simulink model "symbol_mapping"  (R2020b)
settings: Solver=VariableStepAuto  StartTime=0.0  StopTime=10.0  RelTol=1e-3
values from neighbouring files (symbols this model uses):
  fs = 160e6    (= 160000000)    [setup.m]
libraries: hdlsllib x37
settings Model: Creator=ckb13136  LastModifiedBy=LDM

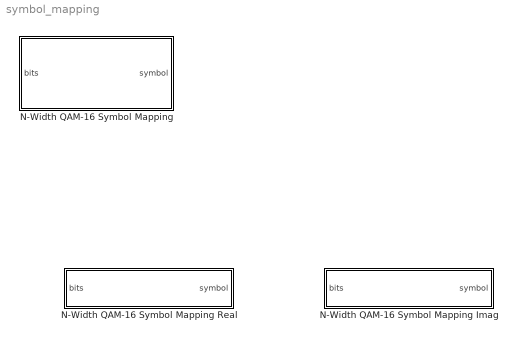
== system symbol_mapping ==
  N-Width QAM-16 Symbol Mapping : Subsystem  mask{bits=4}
      mask prompts: bits "Width:"
      mask init:
      | top_block = gcb;
      | block_names = find_system(top_block, 'LookUnderMasks','on', 'SearchDepth','1');
      | 
      | in_block = sprintf('%s/bits', top_block);
      | out_block = sprintf('%s/symbol', top_block);
      | qam_16_block = sprintf('%s/QAM-16 Symbol Mapping 0', top_block);
      | % enable_block = sprintf('%s/enable', n_qam_16);
      | 
      | keep_blocks = {top_block, in_block, out_block, qam_16_block};
      | 
      | for i = 1:length(block_names)
      |     if ~ismember(block_names{i}, keep_blocks)
      |         delete_block(block_names{i});
      |     end
      | end
      | delete_line(find_system(top_block,'LookUnderMasks', 'all','SearchDepth', '1', 'FindAll','on','type','line'));
      | 
      | % Add QAM-16 Mapping Blocks
      | pos = get_param(qam_16_block, 'position');
      | new_pos = pos;
      | set_param(qam_16_block, 'n', num2str(bits-4));
      | for bit = 4:4:bits-1
      |     new_block = sprintf('%s%d', qam_16_block(1:end-1), bit/4);
      |     add_block(qam_16_block, new_block);
      |     new_pos = pos + ([0 60 0 60] * (bit/4));
      |     set_param(new_block, 'position', new_pos);
      |     set_param(new_block, 'n', num2str(bits-4-bit));
      | end
      | 
      | % Add the Bit Concat
      | concat_block = sprintf('%s/concat', top_block);
      | add_block('hdlsllib/Logic and Bit Operations/Bit Concat', concat_block);
      | set_param(concat_block, 'numInputs', num2str(bits/2));
      | concat_position = new_pos + [175 0 175 0];
      | concat_position(2) = pos(2);
      | set_param(concat_block, 'position', concat_position);
      | 
      | % Reposition Input and Outputs
      | out_position = get_param(out_block, 'position');
      | height = out_position(4) - out_position(2);
      | width = out_position(3) - out_position(1);
      | middle_h = (concat_position(4) - concat_position(2))/2 + concat_position(2);
      | out_position = [concat_position(1) + 175, middle_h - height/2, concat_position(1) + 175 + width, middle_h + height/2];
      | set_param(out_block, 'position', out_position);
      | 
      | in_position = [concat_position(1) - 300, middle_h - height/2, concat_position(1) - 300 + width, middle_h + height/2];
      | set_param(in_block, 'position', in_position);
      | 
      | % enable_position = get_param(enable_block, 'position');
      | % set_param(enable_block, 'position', enable_position - [0 100 0 100]);
      | 
      | % Connect Ports
      | for bit = 1:4:bits
      |     add_line(top_block,'bits/1',sprintf('QAM-16 Symbol Mapping %d/1',(bit-1)/4));
      |     add_line(top_block,sprintf('QAM-16 Symbol Mapping %d/1',(bit-1)/4),sprintf('concat/%d', ceil(bit/2)));
      |     add_line(top_block,sprintf('QAM-16 Symbol Mapping %d/2',(bit-1)/4),sprintf('concat/%d', ceil(bit/2)+1));
      | end
      | add_line(top_block,'concat/1','symbol/1');
  N-Width QAM-16 Symbol Mapping Imag : Subsystem  mask{bits=64}
      mask prompts: bits "Width:"
      mask init:
      | top_block = gcb;
      | set_param(top_block, 'LinkStatus', 'none');
      | 
      | block_names = find_system(top_block, 'LookUnderMasks','on', 'SearchDepth','1');
      | 
      | in_block = sprintf('%s/bits', top_block);
      | out_block = sprintf('%s/symbol', top_block);
      | qam_16_block = sprintf('%s/QAM-16 Symbol Mapping 0', top_block);
      | % enable_block = sprintf('%s/enable', n_qam_16);
      | 
      | keep_blocks = {top_block, in_block, out_block, qam_16_block};
      | 
      | for i = 1:length(block_names)
      |     if ~ismember(block_names{i}, keep_blocks)
      |         delete_block(block_names{i});
      |     end
      | end
      | delete_line(find_system(top_block,'LookUnderMasks', 'all','SearchDepth', '1', 'FindAll','on','type','line'));
      | 
      | % Add QAM-16 Mapping Blocks
      | pos = get_param(qam_16_block, 'position');
      | new_pos = pos;
      | set_param(qam_16_block, 'n', num2str(bits-4));
      | for bit = 4:4:bits-1
      |     new_block = sprintf('%s%d', qam_16_block(1:end-1), bit/4);
      |     add_block(qam_16_block, new_block);
      |     new_pos = pos + ([0 60 0 60] * (bit/4));
      |     set_param(new_block, 'position', new_pos);
      |     set_param(new_block, 'n', num2str(bits-4-bit));
      | end
      | 
      | % Add the Bit Concat
      | concat_block = sprintf('%s/concat', top_block);
      | add_block('hdlsllib/Logic and Bit Operations/Bit Concat', concat_block);
      | set_param(concat_block, 'numInputs', num2str(bits/4));
      | concat_position = new_pos + [175 0 175 0];
      | concat_position(2) = pos(2);
      | set_param(concat_block, 'position', concat_position);
      | 
      | % Reposition Input and Outputs
      | out_position = get_param(out_block, 'position');
      | height = out_position(4) - out_position(2);
      | width = out_position(3) - out_position(1);
      | middle_h = (concat_position(4) - concat_position(2))/2 + concat_position(2);
      | out_position = [concat_position(1) + 175, middle_h - height/2, concat_position(1) + 175 + width, middle_h + height/2];
      | set_param(out_block, 'position', out_position);
      | 
      | in_position = [concat_position(1) - 300, middle_h - height/2, concat_position(1) - 300 + width, middle_h + height/2];
      | set_param(in_block, 'position', in_position);
      | 
      | % enable_position = get_param(enable_block, 'position');
      | % set_param(enable_block, 'position', enable_position - [0 100 0 100]);
      | 
      | % Connect Ports
      | for bit = 1:4:bits
      |     add_line(top_block,'bits/1',sprintf('QAM-16 Symbol Mapping %d/1',(bit-1)/4));
      |     add_line(top_block,sprintf('QAM-16 Symbol Mapping %d/1',(bit-1)/4),sprintf('concat/%d', ceil(bit/4)));
      | %     add_line(top_block,sprintf('QAM-16 Symbol Mapping %d/2',(bit-1)/4),sprintf('concat/%d', ceil(bit/2)+1));
      | end
      | add_line(top_block,'concat/1','symbol/1');
  N-Width QAM-16 Symbol Mapping Real : Subsystem  mask{bits=64}
      mask prompts: bits "Width:"
      mask init: same as symbol_mapping/N-Width QAM-16 Symbol Mapping Imag

== system symbol_mapping/N-Width QAM-16 Symbol Mapping ==
  bits : Inport
  QAM-16 Symbol Mapping 0 : Subsystem  mask{n=0}
  concat : hdlsllib/Logic and Bit Operations/Bit Concat  numInputs=2
  symbol : Outport
  wires:
  bits/1 -> QAM-16 Symbol Mapping 0/1(bits)
  QAM-16 Symbol Mapping 0/1(Q) -> concat/1
  QAM-16 Symbol Mapping 0/2(I) -> concat/2
  concat/1 -> symbol/1

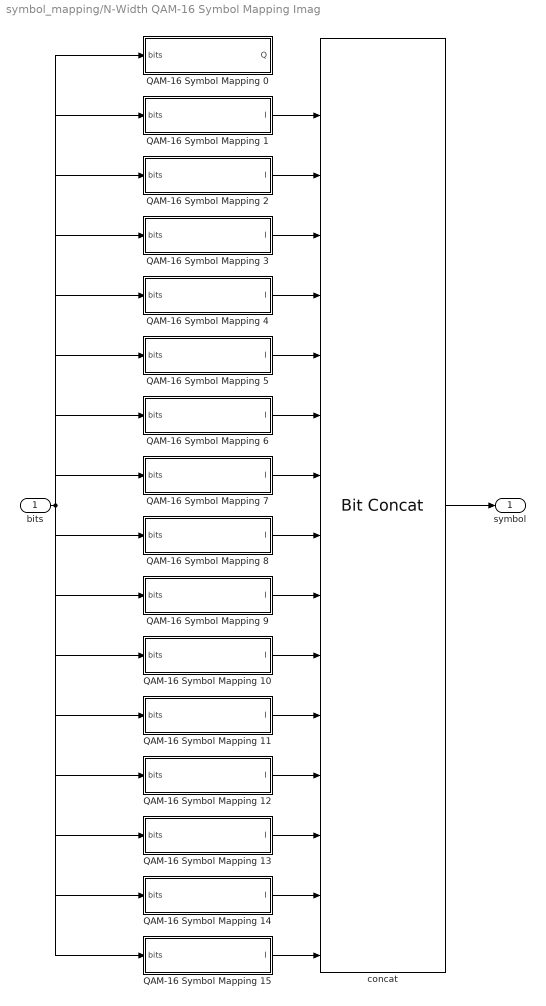
== system symbol_mapping/N-Width QAM-16 Symbol Mapping Imag ==
  bits : Inport
  QAM-16 Symbol Mapping 0 : Subsystem  mask{n=0}
  QAM-16 Symbol Mapping 1 : Subsystem  mask{n=56}
  QAM-16 Symbol Mapping 10 : Subsystem  mask{n=20}
  QAM-16 Symbol Mapping 11 : Subsystem  mask{n=16}
  QAM-16 Symbol Mapping 12 : Subsystem  mask{n=12}
  QAM-16 Symbol Mapping 13 : Subsystem  mask{n=8}
  QAM-16 Symbol Mapping 14 : Subsystem  mask{n=4}
  QAM-16 Symbol Mapping 15 : Subsystem  mask{n=0}
  QAM-16 Symbol Mapping 2 : Subsystem  mask{n=52}
  QAM-16 Symbol Mapping 3 : Subsystem  mask{n=48}
  QAM-16 Symbol Mapping 4 : Subsystem  mask{n=44}
  QAM-16 Symbol Mapping 5 : Subsystem  mask{n=40}
  QAM-16 Symbol Mapping 6 : Subsystem  mask{n=36}
  QAM-16 Symbol Mapping 7 : Subsystem  mask{n=32}
  QAM-16 Symbol Mapping 8 : Subsystem  mask{n=28}
  QAM-16 Symbol Mapping 9 : Subsystem  mask{n=24}
  concat : hdlsllib/Logic and Bit Operations/Bit Concat  numInputs=16
  symbol : Outport
  wires:
  bits/1 -> QAM-16 Symbol Mapping 0/1(bits), QAM-16 Symbol Mapping 1/1(bits), QAM-16 Symbol Mapping 2/1(bits), QAM-16 Symbol Mapping 3/1(bits), QAM-16 Symbol Mapping 4/1(bits), QAM-16 Symbol Mapping 5/1(bits), QAM-16 Symbol Mapping 6/1(bits), QAM-16 Symbol Mapping 7/1(bits), QAM-16 Symbol Mapping 8/1(bits), QAM-16 Symbol Mapping 9/1(bits), QAM-16 Symbol Mapping 10/1(bits), QAM-16 Symbol Mapping 11/1(bits), QAM-16 Symbol Mapping 12/1(bits), QAM-16 Symbol Mapping 13/1(bits), QAM-16 Symbol Mapping 14/1(bits), QAM-16 Symbol Mapping 15/1(bits)
  ? -> concat/1
  QAM-16 Symbol Mapping 1/1(I) -> concat/2
  QAM-16 Symbol Mapping 2/1(I) -> concat/3
  QAM-16 Symbol Mapping 3/1(I) -> concat/4
  QAM-16 Symbol Mapping 4/1(I) -> concat/5
  QAM-16 Symbol Mapping 5/1(I) -> concat/6
  QAM-16 Symbol Mapping 6/1(I) -> concat/7
  QAM-16 Symbol Mapping 7/1(I) -> concat/8
  QAM-16 Symbol Mapping 8/1(I) -> concat/9
  QAM-16 Symbol Mapping 9/1(I) -> concat/10
  QAM-16 Symbol Mapping 10/1(I) -> concat/11
  QAM-16 Symbol Mapping 11/1(I) -> concat/12
  QAM-16 Symbol Mapping 12/1(I) -> concat/13
  QAM-16 Symbol Mapping 13/1(I) -> concat/14
  QAM-16 Symbol Mapping 14/1(I) -> concat/15
  QAM-16 Symbol Mapping 15/1(I) -> concat/16
  concat/1 -> symbol/1

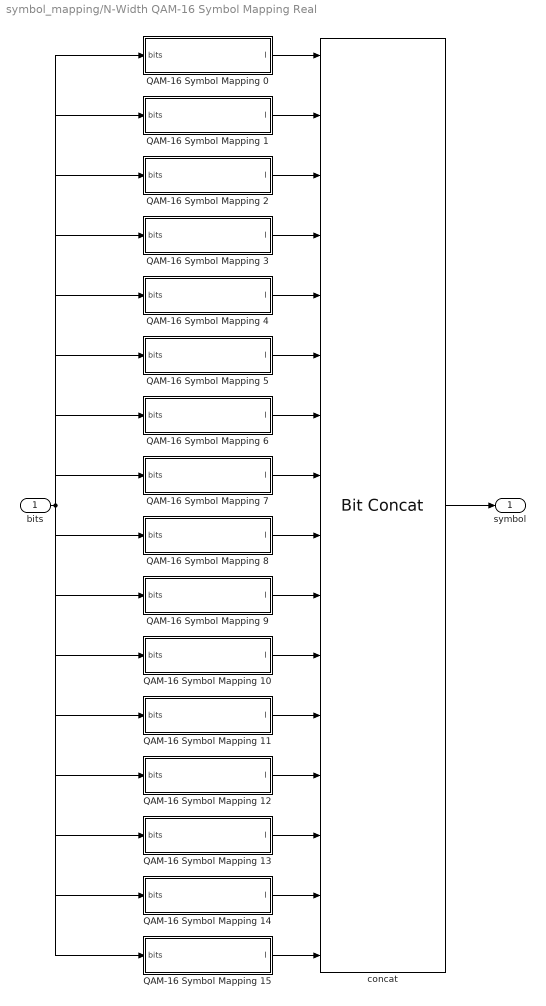
== system symbol_mapping/N-Width QAM-16 Symbol Mapping Real ==
  bits : Inport
  QAM-16 Symbol Mapping 0 : Subsystem  mask{n=60}
  QAM-16 Symbol Mapping 1 : Subsystem  mask{n=56}
  QAM-16 Symbol Mapping 10 : Subsystem  mask{n=20}
  QAM-16 Symbol Mapping 11 : Subsystem  mask{n=16}
  QAM-16 Symbol Mapping 12 : Subsystem  mask{n=12}
  QAM-16 Symbol Mapping 13 : Subsystem  mask{n=8}
  QAM-16 Symbol Mapping 14 : Subsystem  mask{n=4}
  QAM-16 Symbol Mapping 15 : Subsystem  mask{n=0}
  QAM-16 Symbol Mapping 2 : Subsystem  mask{n=52}
  QAM-16 Symbol Mapping 3 : Subsystem  mask{n=48}
  QAM-16 Symbol Mapping 4 : Subsystem  mask{n=44}
  QAM-16 Symbol Mapping 5 : Subsystem  mask{n=40}
  QAM-16 Symbol Mapping 6 : Subsystem  mask{n=36}
  QAM-16 Symbol Mapping 7 : Subsystem  mask{n=32}
  QAM-16 Symbol Mapping 8 : Subsystem  mask{n=28}
  QAM-16 Symbol Mapping 9 : Subsystem  mask{n=24}
  concat : hdlsllib/Logic and Bit Operations/Bit Concat  numInputs=16
  symbol : Outport
  wires:
  bits/1 -> QAM-16 Symbol Mapping 0/1(bits), QAM-16 Symbol Mapping 1/1(bits), QAM-16 Symbol Mapping 2/1(bits), QAM-16 Symbol Mapping 3/1(bits), QAM-16 Symbol Mapping 4/1(bits), QAM-16 Symbol Mapping 5/1(bits), QAM-16 Symbol Mapping 6/1(bits), QAM-16 Symbol Mapping 7/1(bits), QAM-16 Symbol Mapping 8/1(bits), QAM-16 Symbol Mapping 9/1(bits), QAM-16 Symbol Mapping 10/1(bits), QAM-16 Symbol Mapping 11/1(bits), QAM-16 Symbol Mapping 12/1(bits), QAM-16 Symbol Mapping 13/1(bits), QAM-16 Symbol Mapping 14/1(bits), QAM-16 Symbol Mapping 15/1(bits)
  QAM-16 Symbol Mapping 0/1(I) -> concat/1
  QAM-16 Symbol Mapping 1/1(I) -> concat/2
  QAM-16 Symbol Mapping 2/1(I) -> concat/3
  QAM-16 Symbol Mapping 3/1(I) -> concat/4
  QAM-16 Symbol Mapping 4/1(I) -> concat/5
  QAM-16 Symbol Mapping 5/1(I) -> concat/6
  QAM-16 Symbol Mapping 6/1(I) -> concat/7
  QAM-16 Symbol Mapping 7/1(I) -> concat/8
  QAM-16 Symbol Mapping 8/1(I) -> concat/9
  QAM-16 Symbol Mapping 9/1(I) -> concat/10
  QAM-16 Symbol Mapping 10/1(I) -> concat/11
  QAM-16 Symbol Mapping 11/1(I) -> concat/12
  QAM-16 Symbol Mapping 12/1(I) -> concat/13
  QAM-16 Symbol Mapping 13/1(I) -> concat/14
  QAM-16 Symbol Mapping 14/1(I) -> concat/15
  QAM-16 Symbol Mapping 15/1(I) -> concat/16
  concat/1 -> symbol/1

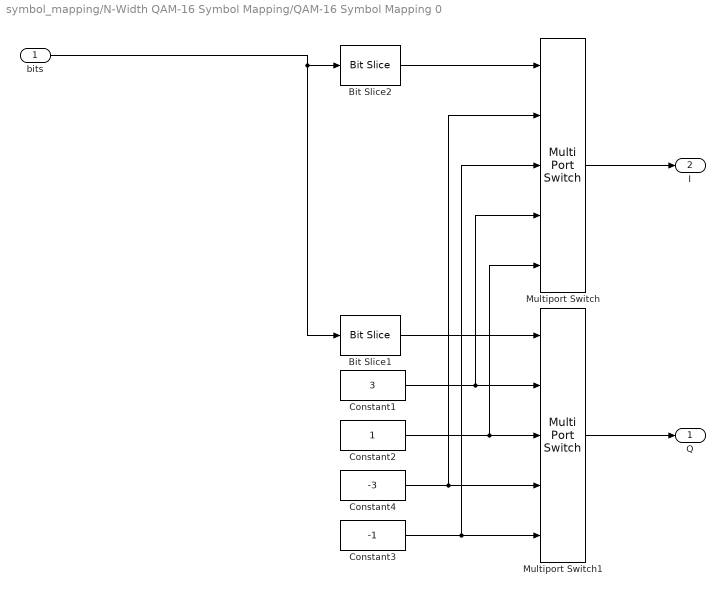
== system symbol_mapping/N-Width QAM-16 Symbol Mapping/QAM-16 Symbol Mapping 0 ==
  bits : Inport
  Bit Slice1 : hdlsllib/Logic and Bit Operations/Bit Slice  lidx=n+1  ridx=n
      settings: SourceProductBaseCode=SL
  Bit Slice2 : hdlsllib/Logic and Bit Operations/Bit Slice  lidx=n+3  ridx=n+2
      settings: SourceProductBaseCode=SL
  Constant1 : Constant  Value=3  OutDataTypeStr=fixdt(1,3,0)  SampleTime=1/(4*fs)
  Constant2 : Constant  OutDataTypeStr=fixdt(1,3,0)  SampleTime=1/(4*fs)
  Constant3 : Constant  Value=-1  OutDataTypeStr=fixdt(1,3,0)  SampleTime=1/(4*fs)
  Constant4 : Constant  Value=-3  OutDataTypeStr=fixdt(1,3,0)  SampleTime=1/(4*fs)
  Multiport Switch : MultiPortSwitch  DataPortOrder=Zero-based contiguous  Inputs=4  zeroidx=on
  Multiport Switch1 : MultiPortSwitch  DataPortOrder=Zero-based contiguous  Inputs=4  zeroidx=on
  Q : Outport
  I : Outport  Port=2
  wires:
  Bit Slice1/1 -> Multiport Switch1/1
  Multiport Switch1/1 -> Q/1
  Bit Slice2/1 -> Multiport Switch/1
  bits/1 -> Bit Slice1/1, Bit Slice2/1
  Constant3/1 -> Multiport Switch/3, Multiport Switch1/5
  Constant4/1 -> Multiport Switch/2, Multiport Switch1/4
  Constant1/1 -> Multiport Switch/4, Multiport Switch1/2
  Constant2/1 -> Multiport Switch/5, Multiport Switch1/3
  Multiport Switch/1 -> I/1

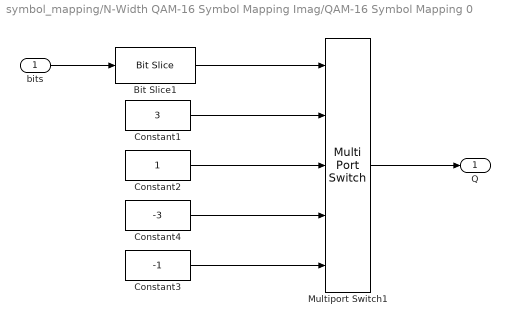
== system symbol_mapping/N-Width QAM-16 Symbol Mapping Imag/QAM-16 Symbol Mapping 0 ==
  bits : Inport
  Bit Slice1 : hdlsllib/Logic and Bit Operations/Bit Slice  lidx=n+1  ridx=n
      settings: SourceProductBaseCode=SL
  Constant1 : Constant  Value=3  OutDataTypeStr=fixdt(1,3,0)  SampleTime=1/(4*fs)
  Constant2 : Constant  OutDataTypeStr=fixdt(1,3,0)  SampleTime=1/(4*fs)
  Constant3 : Constant  Value=-1  OutDataTypeStr=fixdt(1,3,0)  SampleTime=1/(4*fs)
  Constant4 : Constant  Value=-3  OutDataTypeStr=fixdt(1,3,0)  SampleTime=1/(4*fs)
  Multiport Switch1 : MultiPortSwitch  DataPortOrder=Zero-based contiguous  Inputs=4  zeroidx=on
  Q : Outport
  wires:
  Bit Slice1/1 -> Multiport Switch1/1
  Multiport Switch1/1 -> Q/1
  bits/1 -> Bit Slice1/1
  Constant3/1 -> Multiport Switch1/5
  Constant4/1 -> Multiport Switch1/4
  Constant1/1 -> Multiport Switch1/2
  Constant2/1 -> Multiport Switch1/3

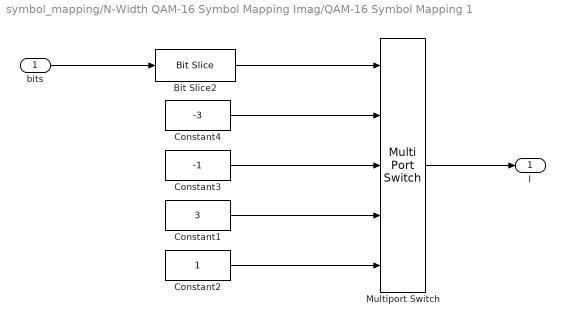
== system symbol_mapping/N-Width QAM-16 Symbol Mapping Imag/QAM-16 Symbol Mapping 1 ==
  bits : Inport
  Bit Slice2 : hdlsllib/Logic and Bit Operations/Bit Slice  lidx=n+3  ridx=n+2
      settings: SourceProductBaseCode=SL
  Constant1 : Constant  Value=3  OutDataTypeStr=fixdt(1,3,0)  SampleTime=-1
  Constant2 : Constant  OutDataTypeStr=fixdt(1,3,0)  SampleTime=-1
  Constant3 : Constant  Value=-1  OutDataTypeStr=fixdt(1,3,0)  SampleTime=-1
  Constant4 : Constant  Value=-3  OutDataTypeStr=fixdt(1,3,0)  SampleTime=-1
  Multiport Switch : MultiPortSwitch  DataPortOrder=Zero-based contiguous  Inputs=4  zeroidx=on
  I : Outport
  wires:
  Bit Slice2/1 -> Multiport Switch/1
  bits/1 -> Bit Slice2/1
  Constant3/1 -> Multiport Switch/3
  Constant4/1 -> Multiport Switch/2
  Constant1/1 -> Multiport Switch/4
  Constant2/1 -> Multiport Switch/5
  Multiport Switch/1 -> I/1

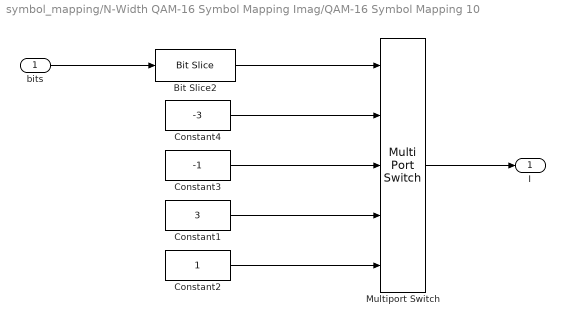
== system symbol_mapping/N-Width QAM-16 Symbol Mapping Imag/QAM-16 Symbol Mapping 10 ==
  bits : Inport
  Bit Slice2 : hdlsllib/Logic and Bit Operations/Bit Slice  lidx=n+3  ridx=n+2
      settings: SourceProductBaseCode=SL
  Constant1 : Constant  Value=3  OutDataTypeStr=fixdt(1,3,0)  SampleTime=-1
  Constant2 : Constant  OutDataTypeStr=fixdt(1,3,0)  SampleTime=-1
  Constant3 : Constant  Value=-1  OutDataTypeStr=fixdt(1,3,0)  SampleTime=-1
  Constant4 : Constant  Value=-3  OutDataTypeStr=fixdt(1,3,0)  SampleTime=-1
  Multiport Switch : MultiPortSwitch  DataPortOrder=Zero-based contiguous  Inputs=4  zeroidx=on
  I : Outport
  wires:
  Bit Slice2/1 -> Multiport Switch/1
  bits/1 -> Bit Slice2/1
  Constant3/1 -> Multiport Switch/3
  Constant4/1 -> Multiport Switch/2
  Constant1/1 -> Multiport Switch/4
  Constant2/1 -> Multiport Switch/5
  Multiport Switch/1 -> I/1

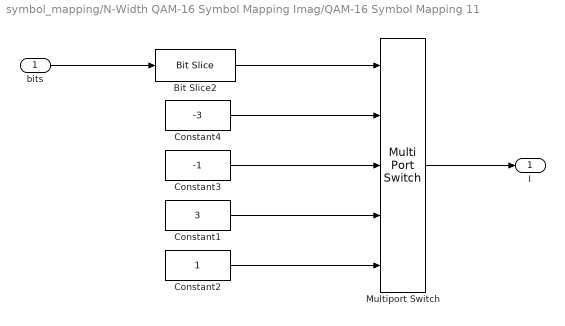
== system symbol_mapping/N-Width QAM-16 Symbol Mapping Imag/QAM-16 Symbol Mapping 11 ==
  bits : Inport
  Bit Slice2 : hdlsllib/Logic and Bit Operations/Bit Slice  lidx=n+3  ridx=n+2
      settings: SourceProductBaseCode=SL
  Constant1 : Constant  Value=3  OutDataTypeStr=fixdt(1,3,0)  SampleTime=-1
  Constant2 : Constant  OutDataTypeStr=fixdt(1,3,0)  SampleTime=-1
  Constant3 : Constant  Value=-1  OutDataTypeStr=fixdt(1,3,0)  SampleTime=-1
  Constant4 : Constant  Value=-3  OutDataTypeStr=fixdt(1,3,0)  SampleTime=-1
  Multiport Switch : MultiPortSwitch  DataPortOrder=Zero-based contiguous  Inputs=4  zeroidx=on
  I : Outport
  wires:
  Bit Slice2/1 -> Multiport Switch/1
  bits/1 -> Bit Slice2/1
  Constant3/1 -> Multiport Switch/3
  Constant4/1 -> Multiport Switch/2
  Constant1/1 -> Multiport Switch/4
  Constant2/1 -> Multiport Switch/5
  Multiport Switch/1 -> I/1

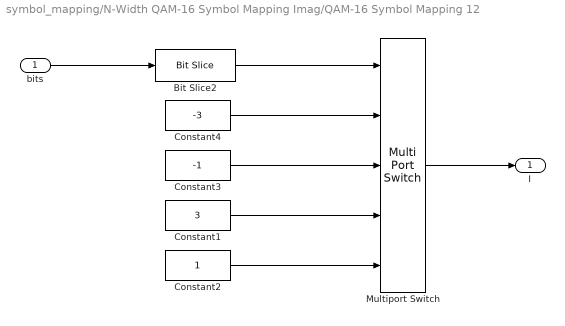
== system symbol_mapping/N-Width QAM-16 Symbol Mapping Imag/QAM-16 Symbol Mapping 12 ==
  bits : Inport
  Bit Slice2 : hdlsllib/Logic and Bit Operations/Bit Slice  lidx=n+3  ridx=n+2
      settings: SourceProductBaseCode=SL
  Constant1 : Constant  Value=3  OutDataTypeStr=fixdt(1,3,0)  SampleTime=-1
  Constant2 : Constant  OutDataTypeStr=fixdt(1,3,0)  SampleTime=-1
  Constant3 : Constant  Value=-1  OutDataTypeStr=fixdt(1,3,0)  SampleTime=-1
  Constant4 : Constant  Value=-3  OutDataTypeStr=fixdt(1,3,0)  SampleTime=-1
  Multiport Switch : MultiPortSwitch  DataPortOrder=Zero-based contiguous  Inputs=4  zeroidx=on
  I : Outport
  wires:
  Bit Slice2/1 -> Multiport Switch/1
  bits/1 -> Bit Slice2/1
  Constant3/1 -> Multiport Switch/3
  Constant4/1 -> Multiport Switch/2
  Constant1/1 -> Multiport Switch/4
  Constant2/1 -> Multiport Switch/5
  Multiport Switch/1 -> I/1

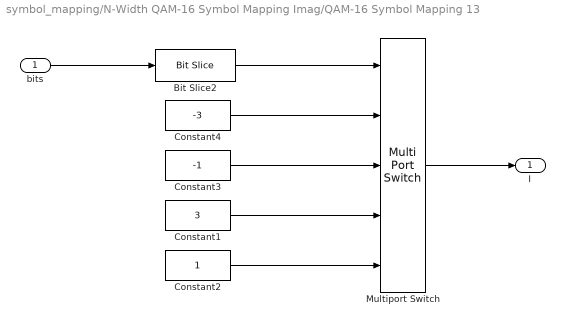
== system symbol_mapping/N-Width QAM-16 Symbol Mapping Imag/QAM-16 Symbol Mapping 13 ==
  bits : Inport
  Bit Slice2 : hdlsllib/Logic and Bit Operations/Bit Slice  lidx=n+3  ridx=n+2
      settings: SourceProductBaseCode=SL
  Constant1 : Constant  Value=3  OutDataTypeStr=fixdt(1,3,0)  SampleTime=-1
  Constant2 : Constant  OutDataTypeStr=fixdt(1,3,0)  SampleTime=-1
  Constant3 : Constant  Value=-1  OutDataTypeStr=fixdt(1,3,0)  SampleTime=-1
  Constant4 : Constant  Value=-3  OutDataTypeStr=fixdt(1,3,0)  SampleTime=-1
  Multiport Switch : MultiPortSwitch  DataPortOrder=Zero-based contiguous  Inputs=4  zeroidx=on
  I : Outport
  wires:
  Bit Slice2/1 -> Multiport Switch/1
  bits/1 -> Bit Slice2/1
  Constant3/1 -> Multiport Switch/3
  Constant4/1 -> Multiport Switch/2
  Constant1/1 -> Multiport Switch/4
  Constant2/1 -> Multiport Switch/5
  Multiport Switch/1 -> I/1

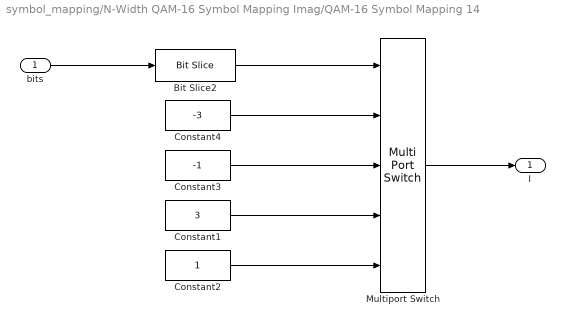
== system symbol_mapping/N-Width QAM-16 Symbol Mapping Imag/QAM-16 Symbol Mapping 14 ==
  bits : Inport
  Bit Slice2 : hdlsllib/Logic and Bit Operations/Bit Slice  lidx=n+3  ridx=n+2
      settings: SourceProductBaseCode=SL
  Constant1 : Constant  Value=3  OutDataTypeStr=fixdt(1,3,0)  SampleTime=-1
  Constant2 : Constant  OutDataTypeStr=fixdt(1,3,0)  SampleTime=-1
  Constant3 : Constant  Value=-1  OutDataTypeStr=fixdt(1,3,0)  SampleTime=-1
  Constant4 : Constant  Value=-3  OutDataTypeStr=fixdt(1,3,0)  SampleTime=-1
  Multiport Switch : MultiPortSwitch  DataPortOrder=Zero-based contiguous  Inputs=4  zeroidx=on
  I : Outport
  wires:
  Bit Slice2/1 -> Multiport Switch/1
  bits/1 -> Bit Slice2/1
  Constant3/1 -> Multiport Switch/3
  Constant4/1 -> Multiport Switch/2
  Constant1/1 -> Multiport Switch/4
  Constant2/1 -> Multiport Switch/5
  Multiport Switch/1 -> I/1

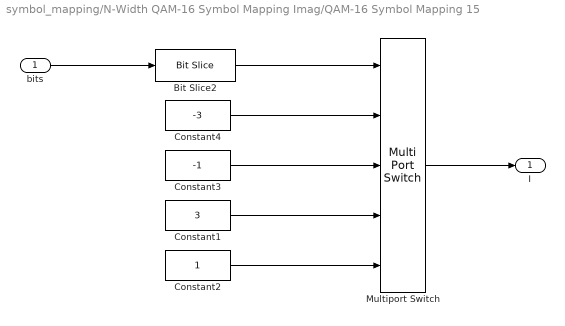
== system symbol_mapping/N-Width QAM-16 Symbol Mapping Imag/QAM-16 Symbol Mapping 15 ==
  bits : Inport
  Bit Slice2 : hdlsllib/Logic and Bit Operations/Bit Slice  lidx=n+3  ridx=n+2
      settings: SourceProductBaseCode=SL
  Constant1 : Constant  Value=3  OutDataTypeStr=fixdt(1,3,0)  SampleTime=-1
  Constant2 : Constant  OutDataTypeStr=fixdt(1,3,0)  SampleTime=-1
  Constant3 : Constant  Value=-1  OutDataTypeStr=fixdt(1,3,0)  SampleTime=-1
  Constant4 : Constant  Value=-3  OutDataTypeStr=fixdt(1,3,0)  SampleTime=-1
  Multiport Switch : MultiPortSwitch  DataPortOrder=Zero-based contiguous  Inputs=4  zeroidx=on
  I : Outport
  wires:
  Bit Slice2/1 -> Multiport Switch/1
  bits/1 -> Bit Slice2/1
  Constant3/1 -> Multiport Switch/3
  Constant4/1 -> Multiport Switch/2
  Constant1/1 -> Multiport Switch/4
  Constant2/1 -> Multiport Switch/5
  Multiport Switch/1 -> I/1

== system symbol_mapping/N-Width QAM-16 Symbol Mapping Imag/QAM-16 Symbol Mapping 2 ==
  bits : Inport
  Bit Slice2 : hdlsllib/Logic and Bit Operations/Bit Slice  lidx=n+3  ridx=n+2
      settings: SourceProductBaseCode=SL
  Constant1 : Constant  Value=3  OutDataTypeStr=fixdt(1,3,0)  SampleTime=-1
  Constant2 : Constant  OutDataTypeStr=fixdt(1,3,0)  SampleTime=-1
  Constant3 : Constant  Value=-1  OutDataTypeStr=fixdt(1,3,0)  SampleTime=-1
  Constant4 : Constant  Value=-3  OutDataTypeStr=fixdt(1,3,0)  SampleTime=-1
  Multiport Switch : MultiPortSwitch  DataPortOrder=Zero-based contiguous  Inputs=4  zeroidx=on
  I : Outport
  wires:
  Bit Slice2/1 -> Multiport Switch/1
  bits/1 -> Bit Slice2/1
  Constant3/1 -> Multiport Switch/3
  Constant4/1 -> Multiport Switch/2
  Constant1/1 -> Multiport Switch/4
  Constant2/1 -> Multiport Switch/5
  Multiport Switch/1 -> I/1

== system symbol_mapping/N-Width QAM-16 Symbol Mapping Imag/QAM-16 Symbol Mapping 3 ==
  bits : Inport
  Bit Slice2 : hdlsllib/Logic and Bit Operations/Bit Slice  lidx=n+3  ridx=n+2
      settings: SourceProductBaseCode=SL
  Constant1 : Constant  Value=3  OutDataTypeStr=fixdt(1,3,0)  SampleTime=-1
  Constant2 : Constant  OutDataTypeStr=fixdt(1,3,0)  SampleTime=-1
  Constant3 : Constant  Value=-1  OutDataTypeStr=fixdt(1,3,0)  SampleTime=-1
  Constant4 : Constant  Value=-3  OutDataTypeStr=fixdt(1,3,0)  SampleTime=-1
  Multiport Switch : MultiPortSwitch  DataPortOrder=Zero-based contiguous  Inputs=4  zeroidx=on
  I : Outport
  wires:
  Bit Slice2/1 -> Multiport Switch/1
  bits/1 -> Bit Slice2/1
  Constant3/1 -> Multiport Switch/3
  Constant4/1 -> Multiport Switch/2
  Constant1/1 -> Multiport Switch/4
  Constant2/1 -> Multiport Switch/5
  Multiport Switch/1 -> I/1

== system symbol_mapping/N-Width QAM-16 Symbol Mapping Imag/QAM-16 Symbol Mapping 4 ==
  bits : Inport
  Bit Slice2 : hdlsllib/Logic and Bit Operations/Bit Slice  lidx=n+3  ridx=n+2
      settings: SourceProductBaseCode=SL
  Constant1 : Constant  Value=3  OutDataTypeStr=fixdt(1,3,0)  SampleTime=-1
  Constant2 : Constant  OutDataTypeStr=fixdt(1,3,0)  SampleTime=-1
  Constant3 : Constant  Value=-1  OutDataTypeStr=fixdt(1,3,0)  SampleTime=-1
  Constant4 : Constant  Value=-3  OutDataTypeStr=fixdt(1,3,0)  SampleTime=-1
  Multiport Switch : MultiPortSwitch  DataPortOrder=Zero-based contiguous  Inputs=4  zeroidx=on
  I : Outport
  wires:
  Bit Slice2/1 -> Multiport Switch/1
  bits/1 -> Bit Slice2/1
  Constant3/1 -> Multiport Switch/3
  Constant4/1 -> Multiport Switch/2
  Constant1/1 -> Multiport Switch/4
  Constant2/1 -> Multiport Switch/5
  Multiport Switch/1 -> I/1

== system symbol_mapping/N-Width QAM-16 Symbol Mapping Imag/QAM-16 Symbol Mapping 5 ==
  bits : Inport
  Bit Slice2 : hdlsllib/Logic and Bit Operations/Bit Slice  lidx=n+3  ridx=n+2
      settings: SourceProductBaseCode=SL
  Constant1 : Constant  Value=3  OutDataTypeStr=fixdt(1,3,0)  SampleTime=-1
  Constant2 : Constant  OutDataTypeStr=fixdt(1,3,0)  SampleTime=-1
  Constant3 : Constant  Value=-1  OutDataTypeStr=fixdt(1,3,0)  SampleTime=-1
  Constant4 : Constant  Value=-3  OutDataTypeStr=fixdt(1,3,0)  SampleTime=-1
  Multiport Switch : MultiPortSwitch  DataPortOrder=Zero-based contiguous  Inputs=4  zeroidx=on
  I : Outport
  wires:
  Bit Slice2/1 -> Multiport Switch/1
  bits/1 -> Bit Slice2/1
  Constant3/1 -> Multiport Switch/3
  Constant4/1 -> Multiport Switch/2
  Constant1/1 -> Multiport Switch/4
  Constant2/1 -> Multiport Switch/5
  Multiport Switch/1 -> I/1

== system symbol_mapping/N-Width QAM-16 Symbol Mapping Imag/QAM-16 Symbol Mapping 6 ==
  bits : Inport
  Bit Slice2 : hdlsllib/Logic and Bit Operations/Bit Slice  lidx=n+3  ridx=n+2
      settings: SourceProductBaseCode=SL
  Constant1 : Constant  Value=3  OutDataTypeStr=fixdt(1,3,0)  SampleTime=-1
  Constant2 : Constant  OutDataTypeStr=fixdt(1,3,0)  SampleTime=-1
  Constant3 : Constant  Value=-1  OutDataTypeStr=fixdt(1,3,0)  SampleTime=-1
  Constant4 : Constant  Value=-3  OutDataTypeStr=fixdt(1,3,0)  SampleTime=-1
  Multiport Switch : MultiPortSwitch  DataPortOrder=Zero-based contiguous  Inputs=4  zeroidx=on
  I : Outport
  wires:
  Bit Slice2/1 -> Multiport Switch/1
  bits/1 -> Bit Slice2/1
  Constant3/1 -> Multiport Switch/3
  Constant4/1 -> Multiport Switch/2
  Constant1/1 -> Multiport Switch/4
  Constant2/1 -> Multiport Switch/5
  Multiport Switch/1 -> I/1

== system symbol_mapping/N-Width QAM-16 Symbol Mapping Imag/QAM-16 Symbol Mapping 7 ==
  bits : Inport
  Bit Slice2 : hdlsllib/Logic and Bit Operations/Bit Slice  lidx=n+3  ridx=n+2
      settings: SourceProductBaseCode=SL
  Constant1 : Constant  Value=3  OutDataTypeStr=fixdt(1,3,0)  SampleTime=-1
  Constant2 : Constant  OutDataTypeStr=fixdt(1,3,0)  SampleTime=-1
  Constant3 : Constant  Value=-1  OutDataTypeStr=fixdt(1,3,0)  SampleTime=-1
  Constant4 : Constant  Value=-3  OutDataTypeStr=fixdt(1,3,0)  SampleTime=-1
  Multiport Switch : MultiPortSwitch  DataPortOrder=Zero-based contiguous  Inputs=4  zeroidx=on
  I : Outport
  wires:
  Bit Slice2/1 -> Multiport Switch/1
  bits/1 -> Bit Slice2/1
  Constant3/1 -> Multiport Switch/3
  Constant4/1 -> Multiport Switch/2
  Constant1/1 -> Multiport Switch/4
  Constant2/1 -> Multiport Switch/5
  Multiport Switch/1 -> I/1

== system symbol_mapping/N-Width QAM-16 Symbol Mapping Imag/QAM-16 Symbol Mapping 8 ==
  bits : Inport
  Bit Slice2 : hdlsllib/Logic and Bit Operations/Bit Slice  lidx=n+3  ridx=n+2
      settings: SourceProductBaseCode=SL
  Constant1 : Constant  Value=3  OutDataTypeStr=fixdt(1,3,0)  SampleTime=-1
  Constant2 : Constant  OutDataTypeStr=fixdt(1,3,0)  SampleTime=-1
  Constant3 : Constant  Value=-1  OutDataTypeStr=fixdt(1,3,0)  SampleTime=-1
  Constant4 : Constant  Value=-3  OutDataTypeStr=fixdt(1,3,0)  SampleTime=-1
  Multiport Switch : MultiPortSwitch  DataPortOrder=Zero-based contiguous  Inputs=4  zeroidx=on
  I : Outport
  wires:
  Bit Slice2/1 -> Multiport Switch/1
  bits/1 -> Bit Slice2/1
  Constant3/1 -> Multiport Switch/3
  Constant4/1 -> Multiport Switch/2
  Constant1/1 -> Multiport Switch/4
  Constant2/1 -> Multiport Switch/5
  Multiport Switch/1 -> I/1

== system symbol_mapping/N-Width QAM-16 Symbol Mapping Imag/QAM-16 Symbol Mapping 9 ==
  bits : Inport
  Bit Slice2 : hdlsllib/Logic and Bit Operations/Bit Slice  lidx=n+3  ridx=n+2
      settings: SourceProductBaseCode=SL
  Constant1 : Constant  Value=3  OutDataTypeStr=fixdt(1,3,0)  SampleTime=-1
  Constant2 : Constant  OutDataTypeStr=fixdt(1,3,0)  SampleTime=-1
  Constant3 : Constant  Value=-1  OutDataTypeStr=fixdt(1,3,0)  SampleTime=-1
  Constant4 : Constant  Value=-3  OutDataTypeStr=fixdt(1,3,0)  SampleTime=-1
  Multiport Switch : MultiPortSwitch  DataPortOrder=Zero-based contiguous  Inputs=4  zeroidx=on
  I : Outport
  wires:
  Bit Slice2/1 -> Multiport Switch/1
  bits/1 -> Bit Slice2/1
  Constant3/1 -> Multiport Switch/3
  Constant4/1 -> Multiport Switch/2
  Constant1/1 -> Multiport Switch/4
  Constant2/1 -> Multiport Switch/5
  Multiport Switch/1 -> I/1

== system symbol_mapping/N-Width QAM-16 Symbol Mapping Real/QAM-16 Symbol Mapping 0 ==
  bits : Inport
  Bit Slice2 : hdlsllib/Logic and Bit Operations/Bit Slice  lidx=n+3  ridx=n+2
      settings: SourceProductBaseCode=SL
  Constant1 : Constant  Value=3  OutDataTypeStr=fixdt(1,3,0)  SampleTime=-1
  Constant2 : Constant  OutDataTypeStr=fixdt(1,3,0)  SampleTime=-1
  Constant3 : Constant  Value=-1  OutDataTypeStr=fixdt(1,3,0)  SampleTime=-1
  Constant4 : Constant  Value=-3  OutDataTypeStr=fixdt(1,3,0)  SampleTime=-1
  Multiport Switch : MultiPortSwitch  DataPortOrder=Zero-based contiguous  Inputs=4  zeroidx=on
  I : Outport
  wires:
  Bit Slice2/1 -> Multiport Switch/1
  bits/1 -> Bit Slice2/1
  Constant3/1 -> Multiport Switch/3
  Constant4/1 -> Multiport Switch/2
  Constant1/1 -> Multiport Switch/4
  Constant2/1 -> Multiport Switch/5
  Multiport Switch/1 -> I/1

== system symbol_mapping/N-Width QAM-16 Symbol Mapping Real/QAM-16 Symbol Mapping 1 ==
  bits : Inport
  Bit Slice2 : hdlsllib/Logic and Bit Operations/Bit Slice  lidx=n+3  ridx=n+2
      settings: SourceProductBaseCode=SL
  Constant1 : Constant  Value=3  OutDataTypeStr=fixdt(1,3,0)  SampleTime=-1
  Constant2 : Constant  OutDataTypeStr=fixdt(1,3,0)  SampleTime=-1
  Constant3 : Constant  Value=-1  OutDataTypeStr=fixdt(1,3,0)  SampleTime=-1
  Constant4 : Constant  Value=-3  OutDataTypeStr=fixdt(1,3,0)  SampleTime=-1
  Multiport Switch : MultiPortSwitch  DataPortOrder=Zero-based contiguous  Inputs=4  zeroidx=on
  I : Outport
  wires:
  Multiport Switch/1 -> I/1
  Constant2/1 -> Multiport Switch/5
  Constant1/1 -> Multiport Switch/4
  Constant4/1 -> Multiport Switch/2
  Constant3/1 -> Multiport Switch/3
  bits/1 -> Bit Slice2/1
  Bit Slice2/1 -> Multiport Switch/1

== system symbol_mapping/N-Width QAM-16 Symbol Mapping Real/QAM-16 Symbol Mapping 10 ==
  bits : Inport
  Bit Slice2 : hdlsllib/Logic and Bit Operations/Bit Slice  lidx=n+3  ridx=n+2
      settings: SourceProductBaseCode=SL
  Constant1 : Constant  Value=3  OutDataTypeStr=fixdt(1,3,0)  SampleTime=-1
  Constant2 : Constant  OutDataTypeStr=fixdt(1,3,0)  SampleTime=-1
  Constant3 : Constant  Value=-1  OutDataTypeStr=fixdt(1,3,0)  SampleTime=-1
  Constant4 : Constant  Value=-3  OutDataTypeStr=fixdt(1,3,0)  SampleTime=-1
  Multiport Switch : MultiPortSwitch  DataPortOrder=Zero-based contiguous  Inputs=4  zeroidx=on
  I : Outport
  wires:
  Multiport Switch/1 -> I/1
  Constant2/1 -> Multiport Switch/5
  Constant1/1 -> Multiport Switch/4
  Constant4/1 -> Multiport Switch/2
  Constant3/1 -> Multiport Switch/3
  bits/1 -> Bit Slice2/1
  Bit Slice2/1 -> Multiport Switch/1

== system symbol_mapping/N-Width QAM-16 Symbol Mapping Real/QAM-16 Symbol Mapping 11 ==
  bits : Inport
  Bit Slice2 : hdlsllib/Logic and Bit Operations/Bit Slice  lidx=n+3  ridx=n+2
      settings: SourceProductBaseCode=SL
  Constant1 : Constant  Value=3  OutDataTypeStr=fixdt(1,3,0)  SampleTime=-1
  Constant2 : Constant  OutDataTypeStr=fixdt(1,3,0)  SampleTime=-1
  Constant3 : Constant  Value=-1  OutDataTypeStr=fixdt(1,3,0)  SampleTime=-1
  Constant4 : Constant  Value=-3  OutDataTypeStr=fixdt(1,3,0)  SampleTime=-1
  Multiport Switch : MultiPortSwitch  DataPortOrder=Zero-based contiguous  Inputs=4  zeroidx=on
  I : Outport
  wires:
  Multiport Switch/1 -> I/1
  Constant2/1 -> Multiport Switch/5
  Constant1/1 -> Multiport Switch/4
  Constant4/1 -> Multiport Switch/2
  Constant3/1 -> Multiport Switch/3
  bits/1 -> Bit Slice2/1
  Bit Slice2/1 -> Multiport Switch/1

== system symbol_mapping/N-Width QAM-16 Symbol Mapping Real/QAM-16 Symbol Mapping 12 ==
  bits : Inport
  Bit Slice2 : hdlsllib/Logic and Bit Operations/Bit Slice  lidx=n+3  ridx=n+2
      settings: SourceProductBaseCode=SL
  Constant1 : Constant  Value=3  OutDataTypeStr=fixdt(1,3,0)  SampleTime=-1
  Constant2 : Constant  OutDataTypeStr=fixdt(1,3,0)  SampleTime=-1
  Constant3 : Constant  Value=-1  OutDataTypeStr=fixdt(1,3,0)  SampleTime=-1
  Constant4 : Constant  Value=-3  OutDataTypeStr=fixdt(1,3,0)  SampleTime=-1
  Multiport Switch : MultiPortSwitch  DataPortOrder=Zero-based contiguous  Inputs=4  zeroidx=on
  I : Outport
  wires:
  Multiport Switch/1 -> I/1
  Constant2/1 -> Multiport Switch/5
  Constant1/1 -> Multiport Switch/4
  Constant4/1 -> Multiport Switch/2
  Constant3/1 -> Multiport Switch/3
  bits/1 -> Bit Slice2/1
  Bit Slice2/1 -> Multiport Switch/1

== system symbol_mapping/N-Width QAM-16 Symbol Mapping Real/QAM-16 Symbol Mapping 13 ==
  bits : Inport
  Bit Slice2 : hdlsllib/Logic and Bit Operations/Bit Slice  lidx=n+3  ridx=n+2
      settings: SourceProductBaseCode=SL
  Constant1 : Constant  Value=3  OutDataTypeStr=fixdt(1,3,0)  SampleTime=-1
  Constant2 : Constant  OutDataTypeStr=fixdt(1,3,0)  SampleTime=-1
  Constant3 : Constant  Value=-1  OutDataTypeStr=fixdt(1,3,0)  SampleTime=-1
  Constant4 : Constant  Value=-3  OutDataTypeStr=fixdt(1,3,0)  SampleTime=-1
  Multiport Switch : MultiPortSwitch  DataPortOrder=Zero-based contiguous  Inputs=4  zeroidx=on
  I : Outport
  wires:
  Multiport Switch/1 -> I/1
  Constant2/1 -> Multiport Switch/5
  Constant1/1 -> Multiport Switch/4
  Constant4/1 -> Multiport Switch/2
  Constant3/1 -> Multiport Switch/3
  bits/1 -> Bit Slice2/1
  Bit Slice2/1 -> Multiport Switch/1

== system symbol_mapping/N-Width QAM-16 Symbol Mapping Real/QAM-16 Symbol Mapping 14 ==
  bits : Inport
  Bit Slice2 : hdlsllib/Logic and Bit Operations/Bit Slice  lidx=n+3  ridx=n+2
      settings: SourceProductBaseCode=SL
  Constant1 : Constant  Value=3  OutDataTypeStr=fixdt(1,3,0)  SampleTime=-1
  Constant2 : Constant  OutDataTypeStr=fixdt(1,3,0)  SampleTime=-1
  Constant3 : Constant  Value=-1  OutDataTypeStr=fixdt(1,3,0)  SampleTime=-1
  Constant4 : Constant  Value=-3  OutDataTypeStr=fixdt(1,3,0)  SampleTime=-1
  Multiport Switch : MultiPortSwitch  DataPortOrder=Zero-based contiguous  Inputs=4  zeroidx=on
  I : Outport
  wires:
  Multiport Switch/1 -> I/1
  Constant2/1 -> Multiport Switch/5
  Constant1/1 -> Multiport Switch/4
  Constant4/1 -> Multiport Switch/2
  Constant3/1 -> Multiport Switch/3
  bits/1 -> Bit Slice2/1
  Bit Slice2/1 -> Multiport Switch/1

== system symbol_mapping/N-Width QAM-16 Symbol Mapping Real/QAM-16 Symbol Mapping 15 ==
  bits : Inport
  Bit Slice2 : hdlsllib/Logic and Bit Operations/Bit Slice  lidx=n+3  ridx=n+2
      settings: SourceProductBaseCode=SL
  Constant1 : Constant  Value=3  OutDataTypeStr=fixdt(1,3,0)  SampleTime=-1
  Constant2 : Constant  OutDataTypeStr=fixdt(1,3,0)  SampleTime=-1
  Constant3 : Constant  Value=-1  OutDataTypeStr=fixdt(1,3,0)  SampleTime=-1
  Constant4 : Constant  Value=-3  OutDataTypeStr=fixdt(1,3,0)  SampleTime=-1
  Multiport Switch : MultiPortSwitch  DataPortOrder=Zero-based contiguous  Inputs=4  zeroidx=on
  I : Outport
  wires:
  Multiport Switch/1 -> I/1
  Constant2/1 -> Multiport Switch/5
  Constant1/1 -> Multiport Switch/4
  Constant4/1 -> Multiport Switch/2
  Constant3/1 -> Multiport Switch/3
  bits/1 -> Bit Slice2/1
  Bit Slice2/1 -> Multiport Switch/1

== system symbol_mapping/N-Width QAM-16 Symbol Mapping Real/QAM-16 Symbol Mapping 2 ==
  bits : Inport
  Bit Slice2 : hdlsllib/Logic and Bit Operations/Bit Slice  lidx=n+3  ridx=n+2
      settings: SourceProductBaseCode=SL
  Constant1 : Constant  Value=3  OutDataTypeStr=fixdt(1,3,0)  SampleTime=-1
  Constant2 : Constant  OutDataTypeStr=fixdt(1,3,0)  SampleTime=-1
  Constant3 : Constant  Value=-1  OutDataTypeStr=fixdt(1,3,0)  SampleTime=-1
  Constant4 : Constant  Value=-3  OutDataTypeStr=fixdt(1,3,0)  SampleTime=-1
  Multiport Switch : MultiPortSwitch  DataPortOrder=Zero-based contiguous  Inputs=4  zeroidx=on
  I : Outport
  wires:
  Multiport Switch/1 -> I/1
  Constant2/1 -> Multiport Switch/5
  Constant1/1 -> Multiport Switch/4
  Constant4/1 -> Multiport Switch/2
  Constant3/1 -> Multiport Switch/3
  bits/1 -> Bit Slice2/1
  Bit Slice2/1 -> Multiport Switch/1

== system symbol_mapping/N-Width QAM-16 Symbol Mapping Real/QAM-16 Symbol Mapping 3 ==
  bits : Inport
  Bit Slice2 : hdlsllib/Logic and Bit Operations/Bit Slice  lidx=n+3  ridx=n+2
      settings: SourceProductBaseCode=SL
  Constant1 : Constant  Value=3  OutDataTypeStr=fixdt(1,3,0)  SampleTime=-1
  Constant2 : Constant  OutDataTypeStr=fixdt(1,3,0)  SampleTime=-1
  Constant3 : Constant  Value=-1  OutDataTypeStr=fixdt(1,3,0)  SampleTime=-1
  Constant4 : Constant  Value=-3  OutDataTypeStr=fixdt(1,3,0)  SampleTime=-1
  Multiport Switch : MultiPortSwitch  DataPortOrder=Zero-based contiguous  Inputs=4  zeroidx=on
  I : Outport
  wires:
  Multiport Switch/1 -> I/1
  Constant2/1 -> Multiport Switch/5
  Constant1/1 -> Multiport Switch/4
  Constant4/1 -> Multiport Switch/2
  Constant3/1 -> Multiport Switch/3
  bits/1 -> Bit Slice2/1
  Bit Slice2/1 -> Multiport Switch/1

== system symbol_mapping/N-Width QAM-16 Symbol Mapping Real/QAM-16 Symbol Mapping 4 ==
  bits : Inport
  Bit Slice2 : hdlsllib/Logic and Bit Operations/Bit Slice  lidx=n+3  ridx=n+2
      settings: SourceProductBaseCode=SL
  Constant1 : Constant  Value=3  OutDataTypeStr=fixdt(1,3,0)  SampleTime=-1
  Constant2 : Constant  OutDataTypeStr=fixdt(1,3,0)  SampleTime=-1
  Constant3 : Constant  Value=-1  OutDataTypeStr=fixdt(1,3,0)  SampleTime=-1
  Constant4 : Constant  Value=-3  OutDataTypeStr=fixdt(1,3,0)  SampleTime=-1
  Multiport Switch : MultiPortSwitch  DataPortOrder=Zero-based contiguous  Inputs=4  zeroidx=on
  I : Outport
  wires:
  Multiport Switch/1 -> I/1
  Constant2/1 -> Multiport Switch/5
  Constant1/1 -> Multiport Switch/4
  Constant4/1 -> Multiport Switch/2
  Constant3/1 -> Multiport Switch/3
  bits/1 -> Bit Slice2/1
  Bit Slice2/1 -> Multiport Switch/1

== system symbol_mapping/N-Width QAM-16 Symbol Mapping Real/QAM-16 Symbol Mapping 5 ==
  bits : Inport
  Bit Slice2 : hdlsllib/Logic and Bit Operations/Bit Slice  lidx=n+3  ridx=n+2
      settings: SourceProductBaseCode=SL
  Constant1 : Constant  Value=3  OutDataTypeStr=fixdt(1,3,0)  SampleTime=-1
  Constant2 : Constant  OutDataTypeStr=fixdt(1,3,0)  SampleTime=-1
  Constant3 : Constant  Value=-1  OutDataTypeStr=fixdt(1,3,0)  SampleTime=-1
  Constant4 : Constant  Value=-3  OutDataTypeStr=fixdt(1,3,0)  SampleTime=-1
  Multiport Switch : MultiPortSwitch  DataPortOrder=Zero-based contiguous  Inputs=4  zeroidx=on
  I : Outport
  wires:
  Multiport Switch/1 -> I/1
  Constant2/1 -> Multiport Switch/5
  Constant1/1 -> Multiport Switch/4
  Constant4/1 -> Multiport Switch/2
  Constant3/1 -> Multiport Switch/3
  bits/1 -> Bit Slice2/1
  Bit Slice2/1 -> Multiport Switch/1

== system symbol_mapping/N-Width QAM-16 Symbol Mapping Real/QAM-16 Symbol Mapping 6 ==
  bits : Inport
  Bit Slice2 : hdlsllib/Logic and Bit Operations/Bit Slice  lidx=n+3  ridx=n+2
      settings: SourceProductBaseCode=SL
  Constant1 : Constant  Value=3  OutDataTypeStr=fixdt(1,3,0)  SampleTime=-1
  Constant2 : Constant  OutDataTypeStr=fixdt(1,3,0)  SampleTime=-1
  Constant3 : Constant  Value=-1  OutDataTypeStr=fixdt(1,3,0)  SampleTime=-1
  Constant4 : Constant  Value=-3  OutDataTypeStr=fixdt(1,3,0)  SampleTime=-1
  Multiport Switch : MultiPortSwitch  DataPortOrder=Zero-based contiguous  Inputs=4  zeroidx=on
  I : Outport
  wires:
  Multiport Switch/1 -> I/1
  Constant2/1 -> Multiport Switch/5
  Constant1/1 -> Multiport Switch/4
  Constant4/1 -> Multiport Switch/2
  Constant3/1 -> Multiport Switch/3
  bits/1 -> Bit Slice2/1
  Bit Slice2/1 -> Multiport Switch/1

== system symbol_mapping/N-Width QAM-16 Symbol Mapping Real/QAM-16 Symbol Mapping 7 ==
  bits : Inport
  Bit Slice2 : hdlsllib/Logic and Bit Operations/Bit Slice  lidx=n+3  ridx=n+2
      settings: SourceProductBaseCode=SL
  Constant1 : Constant  Value=3  OutDataTypeStr=fixdt(1,3,0)  SampleTime=-1
  Constant2 : Constant  OutDataTypeStr=fixdt(1,3,0)  SampleTime=-1
  Constant3 : Constant  Value=-1  OutDataTypeStr=fixdt(1,3,0)  SampleTime=-1
  Constant4 : Constant  Value=-3  OutDataTypeStr=fixdt(1,3,0)  SampleTime=-1
  Multiport Switch : MultiPortSwitch  DataPortOrder=Zero-based contiguous  Inputs=4  zeroidx=on
  I : Outport
  wires:
  Multiport Switch/1 -> I/1
  Constant2/1 -> Multiport Switch/5
  Constant1/1 -> Multiport Switch/4
  Constant4/1 -> Multiport Switch/2
  Constant3/1 -> Multiport Switch/3
  bits/1 -> Bit Slice2/1
  Bit Slice2/1 -> Multiport Switch/1

== system symbol_mapping/N-Width QAM-16 Symbol Mapping Real/QAM-16 Symbol Mapping 8 ==
  bits : Inport
  Bit Slice2 : hdlsllib/Logic and Bit Operations/Bit Slice  lidx=n+3  ridx=n+2
      settings: SourceProductBaseCode=SL
  Constant1 : Constant  Value=3  OutDataTypeStr=fixdt(1,3,0)  SampleTime=-1
  Constant2 : Constant  OutDataTypeStr=fixdt(1,3,0)  SampleTime=-1
  Constant3 : Constant  Value=-1  OutDataTypeStr=fixdt(1,3,0)  SampleTime=-1
  Constant4 : Constant  Value=-3  OutDataTypeStr=fixdt(1,3,0)  SampleTime=-1
  Multiport Switch : MultiPortSwitch  DataPortOrder=Zero-based contiguous  Inputs=4  zeroidx=on
  I : Outport
  wires:
  Multiport Switch/1 -> I/1
  Constant2/1 -> Multiport Switch/5
  Constant1/1 -> Multiport Switch/4
  Constant4/1 -> Multiport Switch/2
  Constant3/1 -> Multiport Switch/3
  bits/1 -> Bit Slice2/1
  Bit Slice2/1 -> Multiport Switch/1

== system symbol_mapping/N-Width QAM-16 Symbol Mapping Real/QAM-16 Symbol Mapping 9 ==
  bits : Inport
  Bit Slice2 : hdlsllib/Logic and Bit Operations/Bit Slice  lidx=n+3  ridx=n+2
      settings: SourceProductBaseCode=SL
  Constant1 : Constant  Value=3  OutDataTypeStr=fixdt(1,3,0)  SampleTime=-1
  Constant2 : Constant  OutDataTypeStr=fixdt(1,3,0)  SampleTime=-1
  Constant3 : Constant  Value=-1  OutDataTypeStr=fixdt(1,3,0)  SampleTime=-1
  Constant4 : Constant  Value=-3  OutDataTypeStr=fixdt(1,3,0)  SampleTime=-1
  Multiport Switch : MultiPortSwitch  DataPortOrder=Zero-based contiguous  Inputs=4  zeroidx=on
  I : Outport
  wires:
  Multiport Switch/1 -> I/1
  Constant2/1 -> Multiport Switch/5
  Constant1/1 -> Multiport Switch/4
  Constant4/1 -> Multiport Switch/2
  Constant3/1 -> Multiport Switch/3
  bits/1 -> Bit Slice2/1
  Bit Slice2/1 -> Multiport Switch/1
